simulink library "Lib_ThermoC_FlowConvertToCan_TMATSC"  (R2019b)
settings: Solver=ode45  StartTime=0.0  StopTime=10.0  RelTol=1e-3  EnableMultiTasking=on
undefined symbols (not defined in the file): comp6_M
Description:
  | Thomas Modules
settings Model: Creator=jwchapm2  LastModifiedBy=bhisma
settings DataIOCC: LimitDataPoints=on  SaveFormat=Array  ReturnWorkspaceOutputs=off
settings OptimizationCC: ExpressionDepthLimit=2147483647  LifeSpan=inf
settings DebuggingCC: UnderspecifiedInitializationDetection=Classic  MergeDetectMultiDrivingBlocksExec=none  SolverPrmCheckMsg=warning  StateNameClashWarn=warning  SFUnexpectedBacktrackingDiag=warning  SFNoUnconditionalDefaultTransitionDiag=warning  SFExecutionAtInitializationDiag=none  ArithmeticOperatorsInVariantConditions=warning
settings HardwareCC: ProdBitPerPointer=32  ProdBitPerSizeT=32  ProdBitPerPtrDiffT=32  ProdLargestAtomicFloat=None  ProdIntDivRoundTo=Undefined  ProdEndianess=Unspecified  ProdWordSize=32  ProdHWDeviceType=32-bit Generic
settings ModelReferenceCC: PropagateSignalLabelsOutOfModel=off
settings SFSimCC: SimUseLocalCustomCode=off  CustomCodeUndefinedFunction=UseInterfaceOnly
settings RTWCC: RTWUseLocalCustomCode=off
settings CodeAppCC: StateflowObjectComments=on
settings GRTTargetCC: TargetLangStandard=C89/C90 (ANSI)  GeneratePreprocessorConditionals=Disable all
settings ConfigComp: CovMetricSettings=dw  CovHtmlReporting=on  CovSaveCumulativeToWorkspaceVar=on  CovSaveSingleToWorkspaceVar=on  CovExternalEMLEnable=off  CovSFcnEnable=off

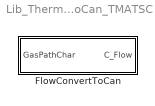
== system Lib_ThermoC_FlowConvertToCan_TMATSC ==
  FlowConvertToCan : Subsystem  mask(TMATS:Flow Convert Library Block, cantera){comp1a_M=1, comp2a_M=0, comp3a_M=0, comp4a_M=0, comp5a_M=0, comp6a_M=0, comp1b_M=1, comp2b_M=0, comp3b_M=0, comp4b_M=0, comp5b_M=0, comp6b_M=0}
      mask prompts: comp1a_M "comp1a_M - species 1 for flow a [weight frac]"; comp2a_M "comp2a_M - species 2 for flow a [weight frac]"; comp3a_M "comp3a_M - species 3 for flow a [weight frac]"; comp4a_M "comp4a_M - species 4 for flow a [weight frac]"; comp5a_M "comp5a_M - species 5 for flow a [weight frac]"; comp6a_M "comp6a_M - species 6 for flow a [weight frac]"; comp1b_M "comp1b_M - species 1 for flow b [weight frac]"; comp2b_M "comp2b_M - species 2 for flow b [weight frac]"; comp3b_M "comp3b_M - species 3 for flow b [weight frac]"; comp4b_M "comp4b_M - species 4 for flow b [weight frac]"; comp5b_M "comp5b_M - species 5 for flow b [weight frac]"; comp6b_M "comp6b_M - species 6 for flow b [weight frac]"
      mask help: This block converts a Gas Path Characterization Bus to a Cantera flow bus.
      mask Help: web(which('ThermoC_TMATSC_FC.html'),'-helpbrowser')
      mask DialogControl Container10 Prompt: Wa
      mask DialogControl Container10_copy Prompt: Wb

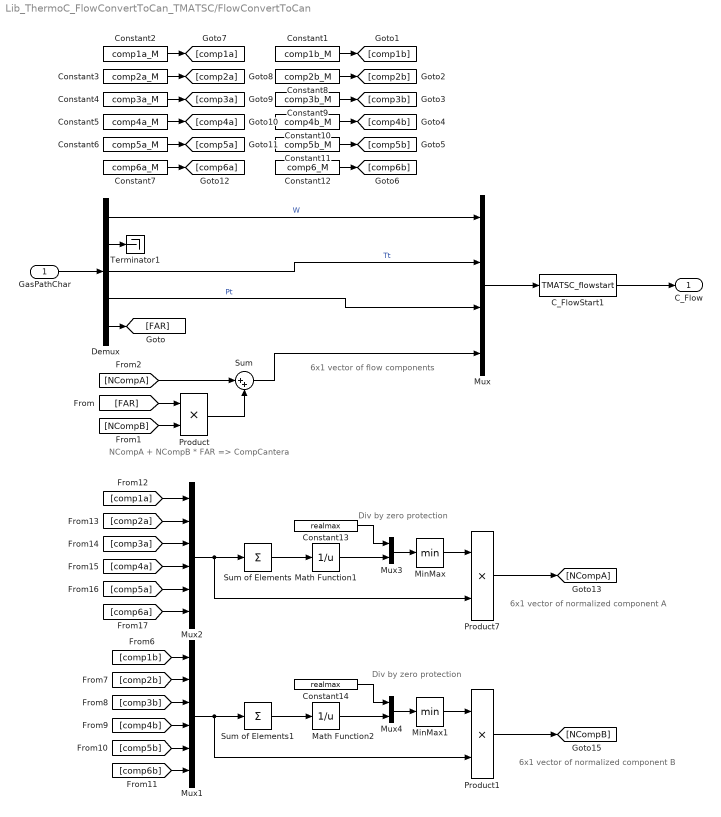
== system Lib_ThermoC_FlowConvertToCan_TMATSC/FlowConvertToCan ==
  note: 6x1 vector of normalized component A
  note: NCompA + NCompB * FAR => CompCantera
  note: 6x1 vector of normalized component B
  note: Div by zero protection
  note: Div by zero protection
  note: 6x1 vector of flow components
  GasPathChar : Inport
  C_FlowStart1 : M-S-Function  FunctionName=TMATSC_flowstart
  Constant1 : Constant  Value=comp1b_M
  Constant10 : Constant  Value=comp4b_M
  Constant11 : Constant  Value=comp5b_M
  Constant12 : Constant  Value=comp6_M
  Constant13 : Constant  Value=realmax
  Constant14 : Constant  Value=realmax
  Constant2 : Constant  Value=comp1a_M
  Constant3 : Constant  Value=comp2a_M
  Constant4 : Constant  Value=comp3a_M
  Constant5 : Constant  Value=comp4a_M
  Constant6 : Constant  Value=comp5a_M
  Constant7 : Constant  Value=comp6a_M
  Constant8 : Constant  Value=comp2b_M
  Constant9 : Constant  Value=comp3b_M
  Demux : Demux  Outputs=5
  Math Function1 : Math  Operator=reciprocal  SaturateOnIntegerOverflow=on
  Math Function2 : Math  Operator=reciprocal  SaturateOnIntegerOverflow=on
  MinMax : MinMax
  MinMax1 : MinMax
  Mux : Mux  Inputs=[1 1 1 6]
  Mux1 : Mux  Inputs=6
  Mux2 : Mux  Inputs=6
  Mux3 : Mux  Inputs=2
  Mux4 : Mux  Inputs=2
  Product : Product
  Product1 : Product
  Product7 : Product
  Sum : Sum  Inputs=|++
  Sum of Elements : Sum  Inputs=+
  Sum of Elements1 : Sum  Inputs=+
  Terminator1 : Terminator
  C_Flow : Outport
  wires:
  C_FlowStart1/1 -> C_Flow/1
  GasPathChar/1 -> Demux/1
  Demux/1 -> Mux/1  "W"
  Demux/3 -> Mux/2  "Tt"
  Demux/4 -> Mux/3  "Pt"
  Demux/5 -> [FAR]
  Demux/2 -> Terminator1/1
  Mux/1 -> C_FlowStart1/1
  Sum/1 -> Mux/4
  [NCompB] -> Product/2
  Product/1 -> Sum/2
  [NCompA] -> Sum/1
  [FAR] -> Product/1
  Constant1/1 -> [comp1b]
  Constant8/1 -> [comp2b]
  Constant9/1 -> [comp3b]
  Constant10/1 -> [comp4b]
  Constant11/1 -> [comp5b]
  Constant12/1 -> [comp6b]
  Constant2/1 -> [comp1a]
  Constant3/1 -> [comp2a]
  Constant4/1 -> [comp3a]
  Constant5/1 -> [comp4a]
  Constant6/1 -> [comp5a]
  Constant7/1 -> [comp6a]
  [comp3b] -> Mux1/3
  [comp2b] -> Mux1/2
  [comp4b] -> Mux1/4
  [comp1b] -> Mux1/1
  [comp5b] -> Mux1/5
  [comp6b] -> Mux1/6
  Mux1/1 -> Product1/2, Sum of Elements1/1
  Sum of Elements1/1 -> Math Function2/1
  [comp1a] -> Mux2/1
  [comp2a] -> Mux2/2
  [comp3a] -> Mux2/3
  [comp4a] -> Mux2/4
  [comp5a] -> Mux2/5
  [comp6a] -> Mux2/6
  Math Function2/1 -> Mux4/2
  Product1/1 -> [NCompB]
  Mux2/1 -> Sum of Elements/1, Product7/2
  Sum of Elements/1 -> Math Function1/1
  Product7/1 -> [NCompA]
  MinMax/1 -> Product7/1
  Math Function1/1 -> Mux3/2
  Mux3/1 -> MinMax/1
  Constant13/1 -> Mux3/1
  Mux4/1 -> MinMax1/1
  MinMax1/1 -> Product1/1
  Constant14/1 -> Mux4/1
